simulink model "linearized_system_state_feedback_spacecraft"  (R2023a)
settings: Solver=VariableStepAuto  StartTime=0.0  StopTime=10  RelTol=1e-3
values from neighbouring files (symbols this model uses):
  A = [0 0 0 1 0 0 ... (first row only)    [linearized_state_space_spacecraft.m]    (also in spacecraft_regulatory_response.m)
  B = [0 0 0 ... (first row only)    [linearized_state_space_spacecraft.m]    (also in spacecraft_regulatory_response.m)
  C = [1 0 0 0 0 0 ... (first row only)    [linearized_state_space_spacecraft.m]    (also in spacecraft_regulatory_response.m)
  K = place(A_bar, B_bar, desired_poles)    [linearized_state_space_spacecraft.m]    (also in spacecraft_regulatory_response.m = place(A, B, desired_poles))
settings Model: Creator=Yogesh  LastModifiedBy=ganes

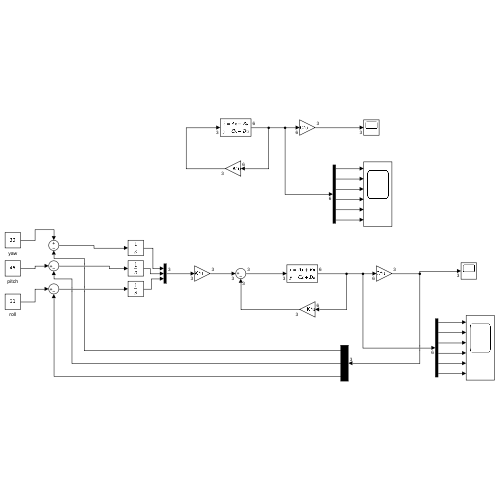
[thumbnail: Simulink's stored preview of the top-level diagram]
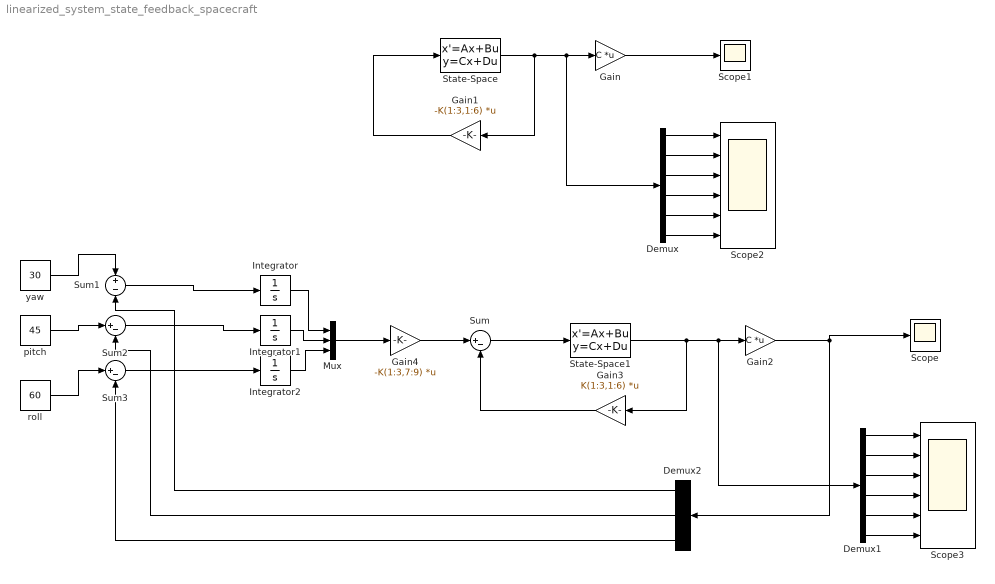
== system linearized_system_state_feedback_spacecraft ==
  Demux : Demux  Outputs=6
  Demux1 : Demux  Outputs=6
  Demux2 : Demux  Outputs=3
  Gain : Gain  Gain=C  Multiplication=Matrix(K*u)
  Gain1 : Gain  Gain=-K(1:3,1:6)  Multiplication=Matrix(K*u)
  Gain2 : Gain  Gain=C  Multiplication=Matrix(K*u)
  Gain3 : Gain  Gain=K(1:3,1:6)  Multiplication=Matrix(K*u)
  Gain4 : Gain  Gain=-K(1:3,7:9)  Multiplication=Matrix(K*u)
  Integrator : Integrator
  Integrator1 : Integrator
  Integrator2 : Integrator
  Mux : Mux  Inputs=3
  Scope : Scope
  Scope1 : Scope
  Scope2 : Scope  NumInputPorts=6
  Scope3 : Scope  NumInputPorts=6
  State-Space : StateSpace  A=A  B=B  C=eye(6)  D=[0 0 0;0 0 0;0 0 0;0 0 0;0 0 0;0 0 0]  InitialCondition=0  ParameterTunability=Unconstrained
  State-Space1 : StateSpace  A=A  B=B  C=eye(6)  D=[0 0 0;0 0 0;0 0 0;0 0 0;0 0 0;0 0 0]  InitialCondition=0  ParameterTunability=Unconstrained
  Sum : Sum  Inputs=|+-
  Sum1 : Sum  Inputs=+-
  Sum2 : Sum  Inputs=|+-
  Sum3 : Sum  Inputs=|+-
  pitch : Constant  Value=45
  roll : Constant  Value=60
  yaw : Constant  Value=30
  wires:
  State-Space/1 -> Demux/1, Gain/1, Gain1/1
  Gain1/1 -> State-Space/1
  Gain/1 -> Scope1/1
  Demux/1 -> Scope2/1
  Demux/4 -> Scope2/4
  Demux/3 -> Scope2/3
  Demux/2 -> Scope2/2
  Demux/5 -> Scope2/5
  Demux/6 -> Scope2/6
  Gain2/1 -> Scope/1, Demux2/1
  Sum/1 -> State-Space1/1
  Gain3/1 -> Sum/2
  Sum1/1 -> Integrator/1
  Sum2/1 -> Integrator1/1
  Sum3/1 -> Integrator2/1
  Gain4/1 -> Sum/1
  Integrator/1 -> Mux/1
  Integrator1/1 -> Mux/2
  Integrator2/1 -> Mux/3
  Mux/1 -> Gain4/1
  yaw/1 -> Sum1/1
  pitch/1 -> Sum2/1
  roll/1 -> Sum3/1
  Demux2/1 -> Sum1/2
  Demux2/2 -> Sum2/2
  Demux2/3 -> Sum3/2
  Demux1/1 -> Scope3/1
  Demux1/2 -> Scope3/2
  Demux1/4 -> Scope3/4
  Demux1/6 -> Scope3/6
  Demux1/3 -> Scope3/3
  Demux1/5 -> Scope3/5
  State-Space1/1 -> Demux1/1, Gain2/1, Gain3/1
